simulink model "LED2"  (R2018b)
settings: Solver=VariableStepAuto  StartTime=0.0  StopTime=10.0  RelTol=1e-3
model workspace (MAT data in the model file):
  V = 5
libraries: fl_lib x5, nesl_utility x5, elec_lib x1
settings Model: Creator=Miodrag Bolic  LastModifiedBy=Miodrag Bolic

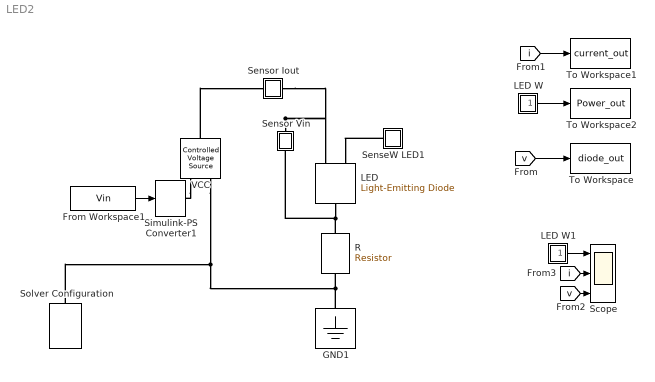
== system LED2 ==
  From Workspace1 : FromWorkspace  VariableName=Vin  SampleTime=0.01  OutputAfterFinalValue=Setting to zero
  GND1 : fl_lib/Electrical/Electrical Elements/Electrical Reference
  LED : elec_lib/Sensors/Light-Emitting Diode  Gain=0.05 W/A  prmExp=1  I12=[.0017, .003] A  V12=[.9, 1.05] V  IS=5e-5 A  ec=10  RS=0.1 Ohm  Tmeas=25 degC  C_param=1  CJ0=20 pF  VJ=1 V  Mgrad=0.5  Vvec=[.1, 10, 100] V  Cvec=[15, 10, 2] pF  FC=0.5  T_param=1  IS_T2=1.8e-4 A  I1_T2=0.0034 A  V1_T2=1.05 V  Tmeas2=125 degC  EG_param=1  EG=1.11 eV  XTI_param=1  XTI=3  Tdevice=25 degC  i_capacitor_specify=off  i_capacitor_priority=High  i_capacitor=0 A  i_capacitor_nominal_specify=off  i_capacitor_nominal_unit=A  i_capacitor_nominal_value=1  v_capacitor_specify=off  v_capacitor_priority=None  v_capacitor=0 V  v_capacitor_nominal_specify=off  v_capacitor_nominal_unit=V  v_capacitor_nominal_value=1  Rth=[0, 10] K/W  thermal_mass_parameterization=1  thermal_mass=[0, 1] J/K  thermal_time_constant=[0, 10] s  thermal_mass_initial_temperatures=[25, 25] degC
      settings: SourceProductName=Simscape Electronics  SourceProductBaseCode=SN
  LED W : Subsystem
  LED W1 : Subsystem
  R : fl_lib/Electrical/Electrical Elements/Resistor  R=0.1 kOhm  i_specify=off  i_priority=None  i=0 A  i_nominal_specify=off  i_nominal_unit=A  i_nominal_value=1  v_specify=off  v_priority=None  v=0 V  v_nominal_specify=off  v_nominal_unit=V  v_nominal_value=1
  Scope : Scope  NumInputPorts=3
  SenseW LED1 : Subsystem
  Sensor Vin : Subsystem
      mask Display: disp('v')
  Sensor Iout : Subsystem
      mask Display: disp('i')
  Simulink-PS Converter1 : nesl_utility/Simulink-PS Converter  PhysicalDomain=network_engine_domain  SubClassName=ps_input  LeftPortType=input  RightPortType=output  PseudoPeriodic=off  Frequencies=[]  NoiseDistribution=none  NoiseParameters=[]  Unit=1  AffineConversion=off  FilteringAndDerivatives=zero  SimscapeFilterOrder=1  InputFilterTimeConstant=0.001  UdotUserProvided=1
  Solver Configuration : nesl_utility/Solver Configuration  PhysicalDomain=network_engine_domain  SubClassName=solver  LeftPortType=input  RightPortType=generic  Tones=[]  Harmonics=[]  SimulateNoise=off  Profile=off  UseLocalSampling=off  EnableSwitchedLinearOptims=on  FrequencyDomain=off  UseCCode=off  RelTol=0.001  AbsTol=1e-06  MinStep=1e-09  ToWorkspace=off  RevertToSquareIcSolve=off  NumHomotopyIterations=100  PhasorMode=off  PhasorModeNumHarmonics=1  DoDC=off  ResidualTolerance=1e-09  UseLocalSolver=off  LocalSolverChoice=NE_BACKWARD_EULER_ADVANCER  LocalSolverSampleTime=0.001  DoFixedCost=off  MaxNonlinIter=3  MaxModeIter=2  LinearAlgebra=Sparse  EquationFormulation=NE_TIME_EF  DelaysMemoryBudget=1024  AutomaticFiltering=on  FilteringTimeConstant=0.001  PartitionStorageMethod=AS_NEEDED  PartitionMemoryBudget=1024
  To Workspace : ToWorkspace  VariableName=diode_out  SaveFormat=Timeseries  SampleTime=-1
  To Workspace1 : ToWorkspace  VariableName=current_out  SaveFormat=Timeseries  SampleTime=-1
  To Workspace2 : ToWorkspace  VariableName=Power_out  SaveFormat=Timeseries  SampleTime=-1
  VCC : fl_lib/Electrical/Electrical Sources/Controlled Voltage Source
  wires:
  [v] -> To Workspace/1
  [i] -> To Workspace1/1
  LED W/1(W) -> To Workspace2/1
  [v] -> Scope/3
  [i] -> Scope/2
  LED W1/1(W) -> Scope/1
  From Workspace1/1 -> Simulink-PS Converter1/1
  connections:
  VCC/RConn2 -- Solver Configuration/RConn1 -- GND1/LConn1 -- R/RConn1
  R/LConn1 -- Sensor Vin/LConn1 -- LED/RConn1
  Sensor Vin/RConn1 -- LED/LConn2 -- Sensor Iout/LConn1
  SenseW LED1/LConn1 -- LED/LConn1
  VCC/LConn1 -- Sensor Iout/RConn1
  VCC/RConn1 -- Simulink-PS Converter1/RConn1

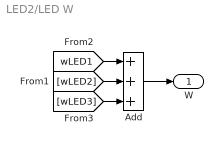
== system LED2/LED W ==
  Add : Sum  Inputs=+++
  W : Outport
  wires:
  Add/1 -> W/1
  [wLED1] -> Add/1
  [wLED2] -> Add/2
  [wLED3] -> Add/3

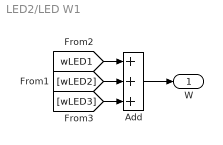
== system LED2/LED W1 ==
  Add : Sum  Inputs=+++
  W : Outport
  wires:
  Add/1 -> W/1
  [wLED1] -> Add/1
  [wLED2] -> Add/2
  [wLED3] -> Add/3

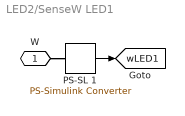
== system LED2/SenseW LED1 ==
  PS-SL 1 : nesl_utility/PS-Simulink Converter  PhysicalDomain=network_engine_domain  SubClassName=ps_output  LeftPortType=input  RightPortType=output  PseudoPeriodic=off  Frequencies=[]  Unit=W  AffineConversion=off
  W : PMIOPort  Side=Left
  tag scope: wLED1=global
  wires:
  PS-SL 1/1 -> [wLED1]
  connections:
  W/RConn1 -- PS-SL 1/LConn1

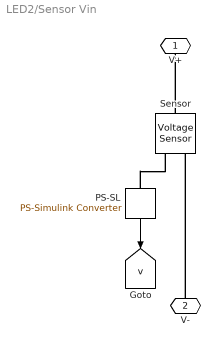
== system LED2/Sensor Vin ==
  PS-SL : nesl_utility/PS-Simulink Converter  PhysicalDomain=network_engine_domain  SubClassName=ps_output  LeftPortType=input  RightPortType=output  PseudoPeriodic=off  Frequencies=[]  Unit=1  AffineConversion=off
  Sensor : fl_lib/Electrical/Electrical Sensors/Voltage Sensor
      settings: SourceProductName=Foundation Library
  V+ : PMIOPort  Side=Right
  V- : PMIOPort  Port=2  Side=Left
  tag scope: v=global
  wires:
  PS-SL/1 -> [v]
  connections:
  PS-SL/LConn1 -- Sensor/RConn1
  Sensor/LConn1 -- V+/RConn1
  V-/RConn1 -- Sensor/RConn2

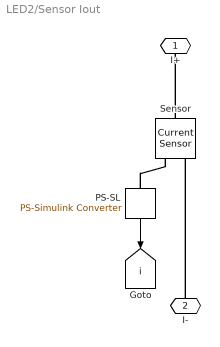
== system LED2/Sensor Iout ==
  PS-SL : nesl_utility/PS-Simulink Converter  PhysicalDomain=network_engine_domain  SubClassName=ps_output  LeftPortType=input  RightPortType=output  PseudoPeriodic=off  Frequencies=[]  Unit=1  AffineConversion=off
  Sensor : fl_lib/Electrical/Electrical Sensors/Current Sensor
      settings: SourceProductName=Foundation Library
  I+ : PMIOPort  Side=Right
  I- : PMIOPort  Port=2  Side=Left
  tag scope: i=global
  wires:
  PS-SL/1 -> [i]
  connections:
  PS-SL/LConn1 -- Sensor/RConn1
  Sensor/LConn1 -- I+/RConn1
  I-/RConn1 -- Sensor/RConn2
